simulink model "gm_ZynqBF_2tx_fpga"  (R2018b)
settings: Solver=FixedStepDiscrete  StartTime=0.0  StopTime=10.0  FixedStep=(1/420e3)/128  RelTol=1e-3
undefined symbols (not defined in the file or in its folder): a, b, c
libraries: hdlsllib x873, simulink x349
(part 5 of 40)

== system gm_ZynqBF_2tx_fpga/channel_estimator/peakdetect_ch1/peak_fsm ==
  t_cross : Inport  OutDataTypeStr=boolean  PortDimensions=1  SampleTime=1.86011904761905e-08
  cnt_end : Inport  Port=2  OutDataTypeStr=boolean  PortDimensions=1  SampleTime=1.86011904761905e-08
  Compare To Constant : simulink/Logic and Bit Operations/Compare To Constant  relop===  const=fi(0,0,8,0,'hex','01')  OutDataTypeStr=boolean
  Compare To Constant1 : simulink/Logic and Bit Operations/Compare To Constant  relop===  const=fi(0,0,8,0,'hex','00')  OutDataTypeStr=boolean
  Compare To Constant2 : simulink/Logic and Bit Operations/Compare To Constant  relop===  const=fi(0,0,8,0,'hex','02')  OutDataTypeStr=boolean
  HDL Counter : hdlsllib/Sources/HDL Counter  CountType=Count limited  CountInit=double(0)  CountStep=double(1)  CountMax=double(3)  CountFromType=Initial value  CountFrom=double(0)  CountResetPort=off  CountLoadPort=off  CountEnbPort=on  CountDirPort=off  CountDataType=Unsigned  CountWordLen=8  CountFracLen=0  CountSampTime=1.86011904761905e-08
      settings: SourceProductBaseCode=HD
  Logical Operator : Logic  AllPortsSameDT=off  OutDataTypeStr=boolean  SampleTime=1.86011904761905e-08
  Logical Operator1 : Logic  Operator=OR  Inputs=3  AllPortsSameDT=off  OutDataTypeStr=boolean  SampleTime=1.86011904761905e-08
  scan_peak : Outport
  peak_found : Outport  Port=2
  wires:
  t_cross/1 -> Logical Operator/1
  cnt_end/1 -> Logical Operator1/2
  Compare To Constant/1 -> scan_peak/1
  Compare To Constant1/1 -> Logical Operator/2
  Compare To Constant2/1 -> Logical Operator1/1, peak_found/1
  HDL Counter/1 -> Compare To Constant2/1, Compare To Constant1/1, Compare To Constant/1
  Logical Operator/1 -> Logical Operator1/3
  Logical Operator1/1 -> HDL Counter/1

== system gm_ZynqBF_2tx_fpga/channel_estimator/peakdetect_ch1/running_max ==
  din : Inport  OutDataTypeStr=fixdt(1, 32, 16)  PortDimensions=1  SampleTime=1.86011904761905e-08
  en : Inport  Port=2  OutDataTypeStr=boolean  PortDimensions=1  SampleTime=1.86011904761905e-08
  rst : Inport  Port=3  OutDataTypeStr=boolean  PortDimensions=1  SampleTime=1.86011904761905e-08
  Constant : Constant  Value=0  OutDataTypeStr=fixdt(1, 32, 16)  SampleTime=-1
  Delay4 : Delay  DelayLength=double(1)  InitialCondition=0  InputProcessing=Inherited  SampleTime=1.86011904761905e-08
  Relational Operator : RelationalOperator  Operator=>  OutDataTypeStr=boolean  SampleTime=1.86011904761905e-08  RndMeth=Nearest
  reset_max : Switch  Criteria=u2 ~= 0  Threshold=double(0)  OutDataTypeStr=fixdt(1, 32, 16)  SampleTime=1.86011904761905e-08
  store_max : Switch  Criteria=u2 ~= 0  Threshold=double(0)  OutDataTypeStr=fixdt(1, 32, 16)  SampleTime=1.86011904761905e-08
  update_max : Logic  AllPortsSameDT=off  OutDataTypeStr=boolean  SampleTime=1.86011904761905e-08
  new_max : Outport
  max_val : Outport  Port=2
  wires:
  din/1 -> store_max/1, Relational Operator/1
  en/1 -> update_max/1
  rst/1 -> reset_max/2
  Constant/1 -> reset_max/1
  Delay4/1 -> store_max/3, Relational Operator/2, max_val/1
  Relational Operator/1 -> update_max/2
  reset_max/1 -> Delay4/1
  store_max/1 -> reset_max/3
  update_max/1 -> store_max/2, new_max/1

== system gm_ZynqBF_2tx_fpga/channel_estimator/peakdetect_ch1/store_index ==
  din : Inport  OutDataTypeStr=int16  PortDimensions=1  SampleTime=1.86011904761905e-08
  update : Inport  Port=2  OutDataTypeStr=boolean  PortDimensions=1  SampleTime=1.86011904761905e-08
  Delay{1..2,4..5} (4 alike) : Delay  DelayLength=double(1)  InitialCondition=0  InputProcessing=Inherited  SampleTime=1.86011904761905e-08
  Switch : Switch  Criteria=u2 ~= 0  Threshold=double(0)  OutDataTypeStr=int16  SampleTime=1.86011904761905e-08
  dout : Outport
  wires:
  din/1 -> Delay2/1
  update/1 -> Delay1/1
  Delay1/1 -> Switch/2
  Delay2/1 -> Switch/1
  Delay4/1 -> dout/1
  Delay5/1 -> Switch/3
  Switch/1 -> Delay5/1, Delay4/1
